simulink model "DCMotorGenset"  (R2021a)
settings: Solver=VariableStepAuto  StartTime=0.0  StopTime=tEnd  RelTol=1e-3
values from neighbouring files (symbols this model uses):
  b = .002    (= 0.002)    [main.m]
  etaGenGR = 0.93    [main.m]
  GRgen = 1.4    [main.m]
  initialGasVolume = 5    [main.m]
  Jm = 5    [main.m]
  k_gal2kWh = 32.3    [main.m]
  k_hr2s = 3600    [main.m]
  k_kW2W = 1000    [main.m]
  k_m32gal = 264.172    [main.m]
  k_rpm2rps = 2*pi()/60    [main.m]
  k_rps2rpm = 60/(2*pi)    (= 9.54929658551)    [main.m]
  k_W2kW = 1/1000    (= 0.001)    [main.m]
  KD_DC = 0.02    [main.m]
  ke = kt    (= 3)    [main.m]
  KI_DC = 0.1    [main.m]
  KP_DC = 5    [main.m]
  kt = 3    [main.m]
  La = .01    (= 0.01)    [main.m]
  motorSpeedCommand = 800    [main.m]
  Ra = .06    (= 0.06)    [main.m]
  torqueCommand = 65    [main.m]
libraries: autolibsharedmappedengines x1, simulink x1
(part 1 of 3)
settings Model: Creator=Chris  LastModifiedBy=jordan
settings SolverCC: AlgebraicLoopSolver=TrustRegion
settings DebuggingCC: SFMachineParentedDataDiag=warning

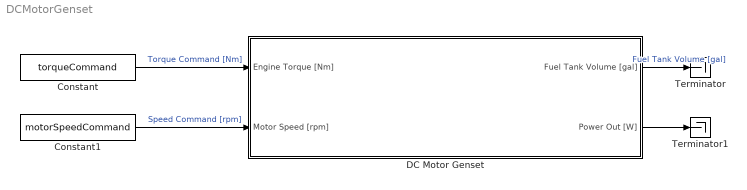
== system DCMotorGenset ==
  Constant : Constant  Value=torqueCommand
  Constant1 : Constant  Value=motorSpeedCommand
  DC Motor Genset : Subsystem
  Terminator : Terminator
  Terminator1 : Terminator
  wires:
  DC Motor Genset/1(Fuel Tank Volume [gal]) -> Terminator/1  "Fuel Tank Volume [gal]"
  DC Motor Genset/2(Power Out [W]) -> Terminator1/1
  Constant/1 -> DC Motor Genset/1(Engine Torque [Nm])  "Torque Command [Nm]"
  Constant1/1 -> DC Motor Genset/2(Motor Speed [rpm])  "Speed Command [rpm]"

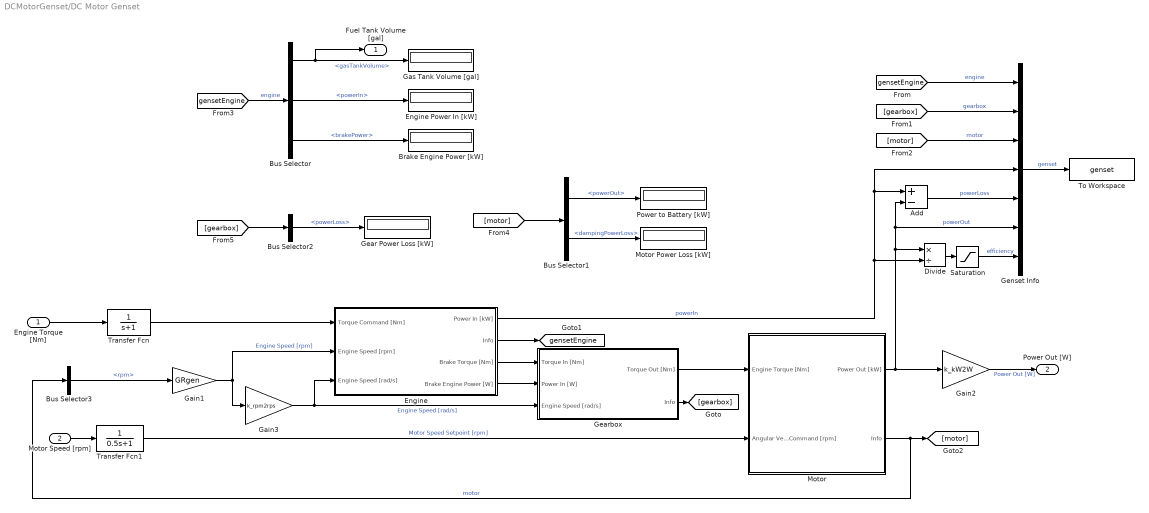
== system DCMotorGenset/DC Motor Genset ==
  Engine Torque [Nm] : Inport
  Motor Speed [rpm] : Inport  Port=2
  Add : Sum  Inputs=+-
  Brake Engine Power [kW] : Display
  Bus Selector : BusSelector  OutputSignals=gasTankVolume,powerIn,brakePower
  Bus Selector1 : BusSelector  OutputSignals=powerOut,dampingPowerLoss
  Bus Selector2 : BusSelector  OutputSignals=powerLoss
  Bus Selector3 : BusSelector  OutputSignals=rpm
  Divide : Product  Inputs=*/
  Engine : Subsystem
  Engine Power In [kW] : Display
  Gain1 : Gain  Gain=GRgen
  Gain2 : Gain  Gain=k_kW2W
  Gain3 : Gain  Gain=k_rpm2rps
  Gas Tank Volume [gal] : Display
  Gear Power Loss [kW] : Display
  Gearbox : Subsystem
  Genset Info : BusCreator  Inputs=7
  Motor : Subsystem
  Motor Power Loss [kW] : Display
  Power to Battery [kW] : Display
  Saturation : Saturate  UpperLimit=1  LowerLimit=0
  To Workspace : ToWorkspace  VariableName=genset  SaveFormat=Timeseries  SampleTime=-1
  Transfer Fcn : TransferFcn  Denominator=[1 1]
  Transfer Fcn1 : TransferFcn  Denominator=[0.5 1]
  Fuel Tank Volume [gal] : Outport
  Power Out [W] : Outport  Port=2
  tag scope: gensetEngine=global
  wires:
  Saturation/1 -> Genset Info/7  "efficiency"
  Bus Selector3/1 -> Gain1/1  "<rpm>"
  Bus Selector1/1 -> Power to Battery [kW]/1  "<powerOut>"
  Add/1 -> Genset Info/5  "powerLoss"
  [gearbox] -> Bus Selector2/1
  Bus Selector/3 -> Brake Engine Power [kW]/1  "<brakePower>"
  [gearbox] -> Genset Info/2  "gearbox"
  [motor] -> Bus Selector1/1
  [gensetEngine] -> Bus Selector/1  "engine"
  Bus Selector/2 -> Engine Power In [kW]/1  "<powerIn>"
  Bus Selector1/2 -> Motor Power Loss [kW]/1  "<dampingPowerLoss>"
  Bus Selector2/1 -> Gear Power Loss [kW]/1  "<powerLoss>"
  Genset Info/1 -> To Workspace/1  "genset"
  Divide/1 -> Saturation/1
  [motor] -> Genset Info/3  "motor"
  [gensetEngine] -> Genset Info/1  "engine"
  Bus Selector/1 -> Gas Tank Volume [gal]/1, Fuel Tank Volume [gal]/1  "<gasTankVolume>"
  Engine/1(Power In [kW]) -> Add/1, Genset Info/4, Divide/2  "powerIn"
  Gain2/1 -> Power Out [W]/1  "Power Out [W]"
  Transfer Fcn/1 -> Engine/1(Torque Command [Nm])
  Engine/4(Brake Engine Power [W]) -> Gearbox/2(Power In [W])
  Engine/2(Info) -> [gensetEngine]
  Gearbox/2(Info) -> [gearbox]
  Motor/1(Power Out [kW]) -> Gain2/1, Divide/1, Genset Info/6, Add/2  "powerOut"
  Gearbox/1(Torque Out [Nm]) -> Motor/1(Engine Torque [Nm])
  Gain3/1 -> Gearbox/3(Engine Speed [rad/s]), Engine/3(Engine Speed [rad/s])  "Engine Speed [rad/s]"
  Engine/3(Brake Torque [Nm]) -> Gearbox/1(Torque In [Nm])
  Transfer Fcn1/1 -> Motor/2(Angular Velocity Command [rpm])  "Motor Speed Setpoint [rpm]"
  Gain1/1 -> Gain3/1, Engine/2(Engine Speed [rpm])  "Engine Speed [rpm]"
  Engine Torque [Nm]/1 -> Transfer Fcn/1
  Motor/2(Info) -> [motor], Bus Selector3/1  "motor"
  Motor Speed [rpm]/1 -> Transfer Fcn1/1
